simulink model "pumps_using_Symhydraulics"  (R2013a)
settings: Solver=ode23tb  StartTime=0.0  StopTime=10.0  RelTol=1e-3
libraries: sh_lib x8, nesl_utility x6, fl_lib x5
settings Model: Creator=Toshiba  LastModifiedBy=Toshiba

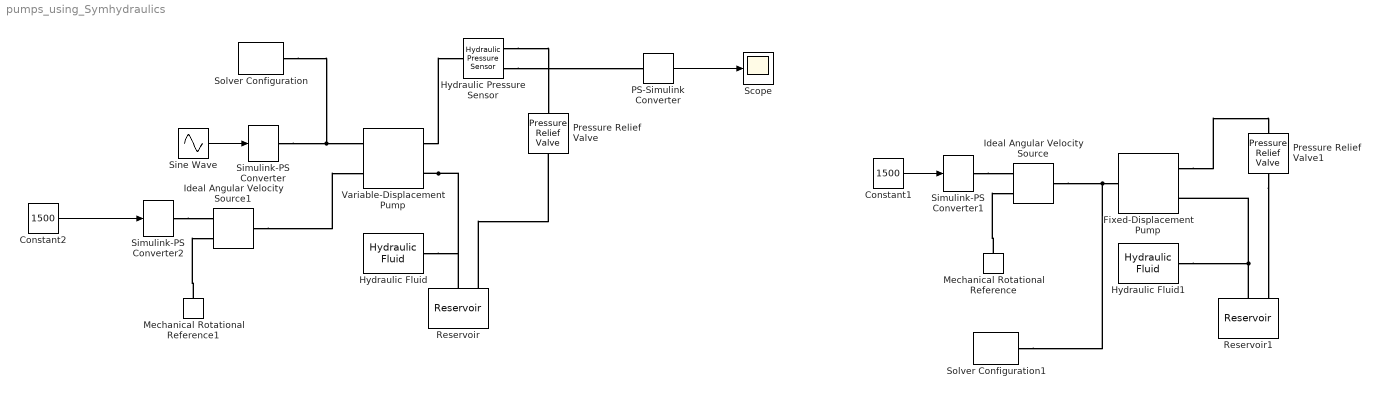
== system pumps_using_Symhydraulics ==
  Constant1 : Constant  Value=1500
  Constant2 : Constant  Value=1500
  Fixed-Displacement Pump : sh_lib/Pumps and Motors/Fixed-Displacement Pump  D=5e-6 m^3/rad  efficiency_vol=0.92  efficiency_tot=0.8  pr_nominal=1e+7 Pa  w_nominal=188 rad/s  visc_nominal=18 cSt  pump_delivery_Log=off  leakage_flow_Log=off  torque_Log=off  power_hyd_Log=off  pressure_diff_Log=off  shaft_ang_vel_Log=off  LocalVarNames=|pump_delivery|leakage_flow|torque|power_hyd|pressure_diff|shaft_ang_vel  LocalVarDescs=|Pump delivery (m^3/s)|Leakage flow rate (m^3/s)|Driving shaft torque (N*m)|Output flow power (W)|Pressure differential (Pa)|Driving shaft angular velocity (rad/s)  LocalVarLogging=[0 0 0 0 0 0]
  Hydraulic Fluid : sh_lib/Hydraulic Utilities/Hydraulic Fluid  DataSource=1  SelFluid=16  SysTemp=60 c  TrapAir=0.001  ViscDerFactor=1  LocalVarLogging=[]
  Hydraulic Fluid1 : sh_lib/Hydraulic Utilities/Hydraulic Fluid  DataSource=1  SelFluid=16  SysTemp=60 c  TrapAir=0.001  ViscDerFactor=1  LocalVarLogging=[]
  Hydraulic Pressure Sensor : fl_lib/Hydraulic/Hydraulic Sensors/Hydraulic Pressure Sensor  q_Log=off  p_Log=off  LocalVarNames=|q|p  LocalVarDescs=|q|p  LocalVarLogging=[0 0]
  Ideal Angular Velocity Source : fl_lib/Mechanical/Mechanical Sources/Ideal Angular Velocity Source  w_Log=off  t_Log=off  LocalVarNames=|w|t  LocalVarDescs=|w|t  LocalVarLogging=[0 0]
  Ideal Angular Velocity Source1 : fl_lib/Mechanical/Mechanical Sources/Ideal Angular Velocity Source  w_Log=off  t_Log=off  LocalVarNames=|w|t  LocalVarDescs=|w|t  LocalVarLogging=[0 0]
  Mechanical Rotational Reference : fl_lib/Mechanical/Rotational Elements/Mechanical Rotational Reference  t_Log=off  LocalVarNames=|t  LocalVarDescs=|t  LocalVarLogging=0
  Mechanical Rotational Reference1 : fl_lib/Mechanical/Rotational Elements/Mechanical Rotational Reference  t_Log=off  LocalVarNames=|t  LocalVarDescs=|t  LocalVarLogging=0
  PS-Simulink Converter : nesl_utility/PS-Simulink Converter  PhysicalDomain=network_engine_domain  SubClassName=ps_output  LeftPortType=input  RightPortType=output  PseudoPeriodic=off  Frequencies=[]  Unit=1  AffineConversion=off
  Pressure Relief Valve : sh_lib/Valves/Pressure Control Valves/Pressure Relief Valve  area_max=1e-4 m^2  pres_set=5e+6 Pa  reg_range=5e+5 Pa  C_d=0.7  Re_cr=12  A_leak=1e-12 m^2  flow_rate_Log=off  pr_drop_Log=off  power_Log=off  area_Log=off  Re_Log=off  LocalVarNames=|flow_rate|pr_drop|power|area|Re  LocalVarDescs=|Flow rate through the valve (m^3/s)|Pressure differential across the valve (Pa)|Hydraulic loss power (W)|Instantaneous passage area (m^2)|Reynolds number  LocalVarLogging=[0 0 0 0 0]
  Pressure Relief Valve1 : sh_lib/Valves/Pressure Control Valves/Pressure Relief Valve  area_max=1e-4 m^2  pres_set=5e+6 Pa  reg_range=5e+5 Pa  C_d=0.7  Re_cr=12  A_leak=1e-12 m^2  flow_rate_Log=off  pr_drop_Log=off  power_Log=off  area_Log=off  Re_Log=off  LocalVarNames=|flow_rate|pr_drop|power|area|Re  LocalVarDescs=|Flow rate through the valve (m^3/s)|Pressure differential across the valve (Pa)|Hydraulic loss power (W)|Instantaneous passage area (m^2)|Reynolds number  LocalVarLogging=[0 0 0 0 0]
  Reservoir : sh_lib/Hydraulic Utilities/Reservoir  press=0 Pa  init_volume=0.02 m^3  ret_diam=0.02 m  loss_coeff=1  fluid_volume_Log=off  flow_rate_ret_Log=off  flow_rate_tank_Log=off  pr_loss_ret_Log=off  power_loss_Log=off  LocalVarNames=|fluid_volume|flow_rate_ret|flow_rate_tank|pr_loss_ret|power_loss  LocalVarDescs=|Fluid volume (m^3)|Flow rate in return line (m^3/s)|Flow rate into tank (m^3/s)|Pressure loss in return line (Pa)|Power loss in return line (Pa)  LocalVarLogging=[0 0 0 0 0]
  Reservoir1 : sh_lib/Hydraulic Utilities/Reservoir  press=0 Pa  init_volume=0.02 m^3  ret_diam=0.02 m  loss_coeff=1  fluid_volume_Log=off  flow_rate_ret_Log=off  flow_rate_tank_Log=off  pr_loss_ret_Log=off  power_loss_Log=off  LocalVarNames=|fluid_volume|flow_rate_ret|flow_rate_tank|pr_loss_ret|power_loss  LocalVarDescs=|Fluid volume (m^3)|Flow rate in return line (m^3/s)|Flow rate into tank (m^3/s)|Pressure loss in return line (Pa)|Power loss in return line (Pa)  LocalVarLogging=[0 0 0 0 0]
  Scope : Scope
  Simulink-PS Converter : nesl_utility/Simulink-PS Converter  PhysicalDomain=network_engine_domain  SubClassName=ps_input  LeftPortType=input  RightPortType=output  PseudoPeriodic=off  Frequencies=[]  NoiseDistribution=none  NoiseParameters=[]  Unit=1  AffineConversion=off  InputFiltering=on  SimscapeFilterOrder=1  InputFilterTimeConstant=0.001  UdotUserProvided=1
  Simulink-PS Converter1 : nesl_utility/Simulink-PS Converter  PhysicalDomain=network_engine_domain  SubClassName=ps_input  LeftPortType=input  RightPortType=output  PseudoPeriodic=off  Frequencies=[]  NoiseDistribution=none  NoiseParameters=[]  Unit=1  AffineConversion=off  InputFiltering=off  SimscapeFilterOrder=1  InputFilterTimeConstant=0.001  UdotUserProvided=1
  Simulink-PS Converter2 : nesl_utility/Simulink-PS Converter  PhysicalDomain=network_engine_domain  SubClassName=ps_input  LeftPortType=input  RightPortType=output  PseudoPeriodic=off  Frequencies=[]  NoiseDistribution=none  NoiseParameters=[]  Unit=1  AffineConversion=off  InputFiltering=off  SimscapeFilterOrder=1  InputFilterTimeConstant=0.001  UdotUserProvided=1
  Sine Wave : Sin  Amplitude=0.5  SampleTime=0
  Solver Configuration : nesl_utility/Solver Configuration  PhysicalDomain=network_engine_domain  SubClassName=solver  LeftPortType=input  RightPortType=generic  Accelerate=off  Tones=[]  Harmonics=[]  SimulateNoise=off  Profile=off  UseLocalSampling=off  EnableSwitchedLinearOptims=on  FrequencyDomain=off  UseCCode=off  UseNewInitialization=off  DoDC=off  ResidualTolerance=1e-09  UseLocalSolver=on  LocalSolverChoice=NE_TRAPEZOIDAL_ADVANCER  LocalSolverSampleTime=0.001  DoFixedCost=on  MaxNonlinIter=3  MaxModeIter=2  LinearAlgebra=Sparse  DelaysMemoryBudget=1024
  Solver Configuration1 : nesl_utility/Solver Configuration  PhysicalDomain=network_engine_domain  SubClassName=solver  LeftPortType=input  RightPortType=generic  Accelerate=off  Tones=[]  Harmonics=[]  SimulateNoise=off  Profile=off  UseLocalSampling=off  EnableSwitchedLinearOptims=on  FrequencyDomain=off  UseCCode=off  UseNewInitialization=off  DoDC=off  ResidualTolerance=1e-09  UseLocalSolver=on  LocalSolverChoice=NE_TRAPEZOIDAL_ADVANCER  LocalSolverSampleTime=0.001  DoFixedCost=on  MaxNonlinIter=3  MaxModeIter=2  LinearAlgebra=Sparse  DelaysMemoryBudget=1024
  Variable-Displacement Pump : sh_lib/Pumps and Motors/Variable-Displacement Pump  mdl_type=1  D_max=5e-6 m^3/rad  stroke_max=0.005 m  cntrl_mem_tab=[ -0.0075 -0.0025 0 0.0025 0.0075 ] m  displ_tab=[ -5e-6 -3e-6 0 3e-6 5e-6 ] m^3/rad  interp_method=1  extrap_method=1  efficiency_vol=0.85  efficiency_tot=0.75  pr_nominal=1e+7 Pa  w_nominal=188 rad/s  visc_nominal=18 cSt  pump_delivery_Log=off  pr_drop_Log=off  leakage_flow_Log=off  torque_Log=off  ang_velocity_Log=off  displacement_Log=off  power_hyd_Log=off  LocalVarNames=|pump_delivery|pr_drop|leakage_flow|torque|ang_velocity|displacement|power_hyd  LocalVarDescs=|Pump delivery (m^3/s)|Pressure differential across the pump (Pa)|Leakage flow rate (m^3/s)|Driving shaft torque (N*m)|Driving shaft angular velocity (rad/s)|Pump displacement (m^3/rad)|Output flow power (W)  LocalVarLogging=[0 0 0 0 0 0 0]
  wires:
  Sine Wave/1 -> Simulink-PS Converter/1
  Constant1/1 -> Simulink-PS Converter1/1
  Constant2/1 -> Simulink-PS Converter2/1
  PS-Simulink Converter/1 -> Scope/1
  connections:
  Variable-Displacement Pump/RConn2 -- Reservoir/LConn2 -- Hydraulic Fluid/RConn1
  Fixed-Displacement Pump/RConn1 -- Pressure Relief Valve1/LConn1
  Pressure Relief Valve1/RConn1 -- Reservoir1/LConn3
  Reservoir1/LConn2 -- Hydraulic Fluid1/RConn1 -- Fixed-Displacement Pump/RConn2
  Simulink-PS Converter/RConn1 -- Solver Configuration/RConn1 -- Variable-Displacement Pump/LConn1
  Ideal Angular Velocity Source/LConn1 -- Fixed-Displacement Pump/LConn1 -- Solver Configuration1/RConn1
  Simulink-PS Converter1/RConn1 -- Ideal Angular Velocity Source/RConn1
  Mechanical Rotational Reference/LConn1 -- Ideal Angular Velocity Source/RConn2
  Simulink-PS Converter2/RConn1 -- Ideal Angular Velocity Source1/RConn1
  Mechanical Rotational Reference1/LConn1 -- Ideal Angular Velocity Source1/RConn2
  Ideal Angular Velocity Source1/LConn1 -- Variable-Displacement Pump/LConn2
  Hydraulic Pressure Sensor/RConn2 -- PS-Simulink Converter/LConn1
  Variable-Displacement Pump/RConn1 -- Hydraulic Pressure Sensor/LConn1
  Hydraulic Pressure Sensor/RConn1 -- Pressure Relief Valve/LConn1
  Reservoir/LConn3 -- Pressure Relief Valve/RConn1
